simulink model "Inverter1"  (R2013a)
settings: Solver=ode45  StartTime=0.0  StopTime=1  RelTol=1e-3
libraries: powerlib x19, simulink x1
settings Model: Creator=HP6k  LastModifiedBy=HP6k

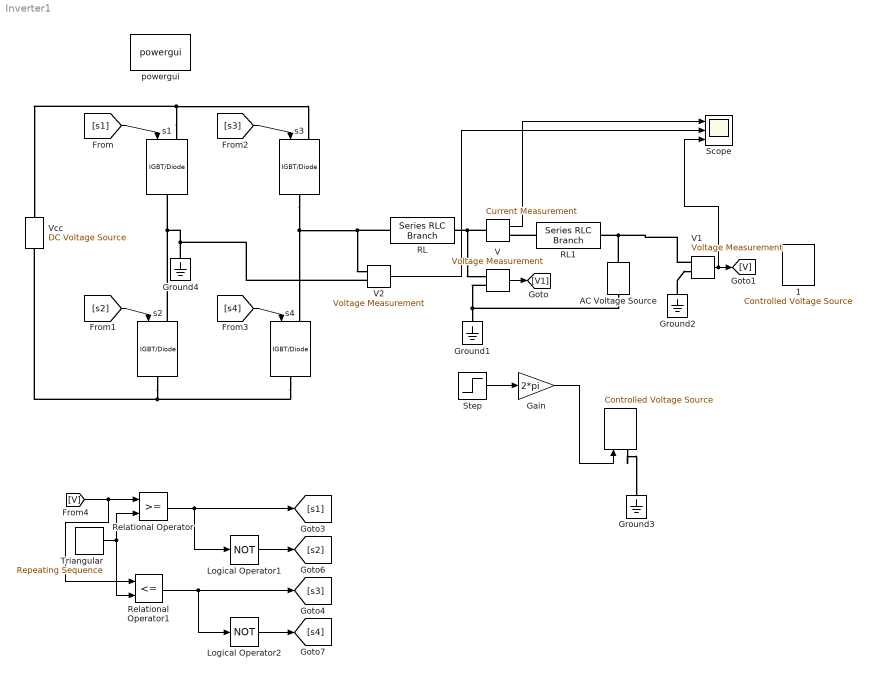
== system Inverter1 ==
  " " : powerlib/Measurements/Current Measurement  PhasorSimulation=off  OutputType=Complex  PSBequivalent=0
  " " : powerlib/Electrical Sources/Controlled Voltage Source  Initialize=on  Source_Type=AC  Amplitude=311  Phase=0  Frequency=50  Measurements=None
  " 1" : powerlib/Electrical Sources/Controlled Voltage Source  Initialize=on  Source_Type=AC  Amplitude=0  Phase=0  Frequency=0  Measurements=None
  AC Voltage Source : powerlib/Electrical Sources/AC Voltage Source  Amplitude=311  Phase=0  Frequency=50  SampleTime=0  Measurements=None
  Gain : Gain  Gain=2*pi
  Ground{1..4} (4 alike) : powerlib/Elements/Ground  LConnTagsString=a
  Logical Operator1 : Logic  Operator=NOT  AllPortsSameDT=off  OutDataTypeStr=boolean
  Logical Operator2 : Logic  Operator=NOT  AllPortsSameDT=off  OutDataTypeStr=boolean
  RL : powerlib/Elements/Series RLC Branch  LConnTagsString=__new0  RConnTagsString=__new0  BranchType=RL  Resistance=1  Inductance=1e-3  SetiL0=off  InitialCurrent=0  Capacitance=1e-6  Setx0=off  InitialVoltage=0  Measurements=None
  RL1 : powerlib/Elements/Series RLC Branch  LConnTagsString=__new0  RConnTagsString=__new0  BranchType=RL  Resistance=1  Inductance=1e-3  SetiL0=off  InitialCurrent=0  Capacitance=1e-6  Setx0=off  InitialVoltage=0  Measurements=None
  Relational Operator : RelationalOperator  OutDataTypeStr=boolean
  Relational Operator1 : RelationalOperator  Operator=<=  OutDataTypeStr=boolean
  Scope : Scope  NumInputPorts=3
      settings: TimeRange=0.006000000000000005  YMin=-200~-400~-350  YMax=-60~300~50
  Step : Step  Before=50  After=50  SampleTime=0
  Triangular : simulink/Sources/Repeating Sequence  rep_seq_t=[0 0.5 1]*1/10E3  rep_seq_y=[-1 1 -1]
  V : powerlib/Measurements/Voltage Measurement  PhasorSimulation=off  OutputType=Complex  PSBequivalent=0
  V1 : powerlib/Measurements/Voltage Measurement  PhasorSimulation=off  OutputType=Complex  PSBequivalent=0
  V2 : powerlib/Measurements/Voltage Measurement  PhasorSimulation=off  OutputType=Complex  PSBequivalent=0
  Vcc : powerlib/Electrical Sources/DC Voltage Source  Amplitude=450  Measurements=None
  powergui : powerlib/powergui  Priority=1  SimulationMode=Discrete  SolverType=Tustin  SampleTime=1e-6  frequency=60  SPID=off  DisableSnubberDevices=off  DisableRonSwitches=off  DisableVfSwitches=off  SwTol=0  Interpol=off  DisplayEquations=off  frequencyindice=50  Pbase=100e6  ErrMax=1e-4  Iterations=50  UnitsV=kV  UnitsW=MW  FunctionMessages=off  echomessages=off  HookPort=off  EnableUseOfTLC=off  x0status=blocks  RestoreLinks=warning  ResistiveCurrentMeasurement=off  Frange=[0:2:500]  Ylog=off  Xlog=on  ShowGrid=off  save=off  variable=ZData  ZoomFFT=off  StartTime=0.0  cycles=1  DisplayStyle=1  fundamental=60  FreqAxis=off  MaxFrequency=1000  frequencyindicesteady=1  RmsSteady=1  display=off  Ts=0  methode=off
  s{1..4} (4 alike) : powerlib/Power Electronics/IGBT//Diode  Ron=1e-4  Rs=1e5  Cs=inf  Measurements=off
  wires:
  [s1] -> s1/1
  [s3] -> s3/1
  [s4] -> s4/1
  [s2] -> s2/1
  Relational Operator/1 -> Logical Operator1/1, [s1]
  Logical Operator1/1 -> [s2]
  Triangular/1 -> Relational Operator1/2, Relational Operator/2
  Logical Operator2/1 -> [s4]
  Relational Operator1/1 -> [s3], Logical Operator2/1
  [V] -> Relational Operator1/1, Relational Operator/1
  V/1 -> [V1]
  V1/1 -> Scope/3, [V]
  Step/1 -> Gain/1
  Gain/1 -> " "/1
  " "/1 -> Scope/1
  V2/1 -> Scope/2
  connections:
  s3/RConn1 -- s4/LConn1 -- V2/LConn1 -- RL/LConn1
  s4/RConn1 -- Vcc/LConn1 -- s2/RConn1
  s1/LConn1 -- s3/LConn1 -- Vcc/RConn1
  RL/RConn1 -- V/LConn1 -- " "/LConn1
  RL1/LConn1 -- " "/RConn1
  V1/LConn1 -- AC Voltage Source/RConn1 -- RL1/RConn1
  V/LConn2 -- AC Voltage Source/LConn1 -- Ground1/LConn1
  Ground2/LConn1 -- V1/LConn2
  " "/LConn1 -- Ground3/LConn1
  s2/LConn1 -- V2/LConn2 -- Ground4/LConn1 -- s1/RConn1
